simulink model "exercise_04_09_fbk_block"  (R2020a)
settings: Solver=VariableStepAuto  StartTime=0.0  StopTime=10.0  RelTol=1e-3
settings Model: Creator=kawata  LastModifiedBy=kawata

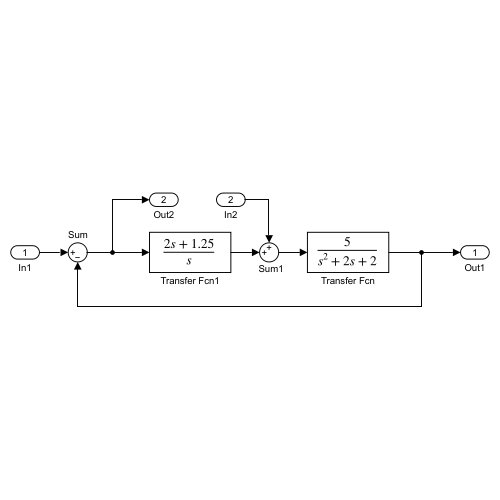
[thumbnail: Simulink's stored preview of the top-level diagram]
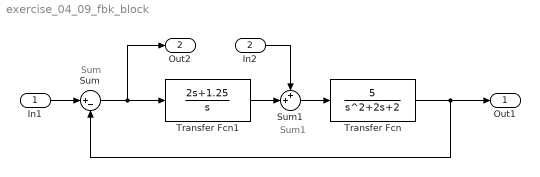
== system exercise_04_09_fbk_block ==
  note: Sum
  note: Sum1
  In1 : Inport
  In2 : Inport  Port=2
  Sum : Sum  Inputs=|+-
  Sum1 : Sum  Inputs=++|
  Transfer Fcn : TransferFcn  Numerator=[5]  Denominator=[1 2 2]
  Transfer Fcn1 : TransferFcn  Numerator=[2 1.25]  Denominator=[1 0]
  Out1 : Outport
  Out2 : Outport  Port=2
  wires:
  In1/1 -> Sum/1
  Sum/1 -> Transfer Fcn1/1, Out2/1
  Transfer Fcn1/1 -> Sum1/2
  In2/1 -> Sum1/1
  Sum1/1 -> Transfer Fcn/1
  Transfer Fcn/1 -> Out1/1, Sum/2
